simulink model "train_model_PetrFD"  (R2021b)
settings: Solver=FixedStepAuto  StartTime=0.0  StopTime=10  FixedStep=0.01  RelTol=1e-3
model workspace (MAT data in the model file):
  L = 50
  g = 9.8
undefined symbols (not defined in the file): l
libraries: simulink_extras x2
settings Model: Creator=PC  LastModifiedBy=PC

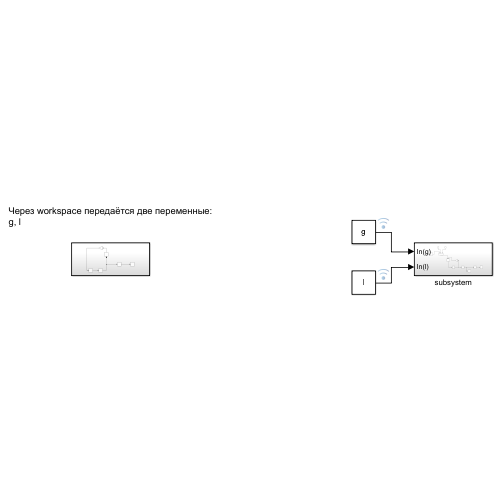
[thumbnail: Simulink's stored preview of the top-level diagram]
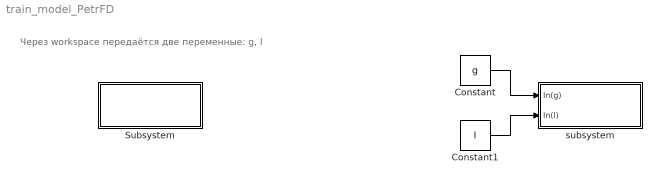
== system train_model_PetrFD ==
  note: Через workspace передаётся две переменные:
      | g, l
  Constant : Constant  Value=g
  Constant1 : Constant  Value=l
  Subsystem : Subsystem
  subsystem : Subsystem
  wires:
  Constant/1 -> subsystem/1(In(g))
  Constant1/1 -> subsystem/2(In(l))

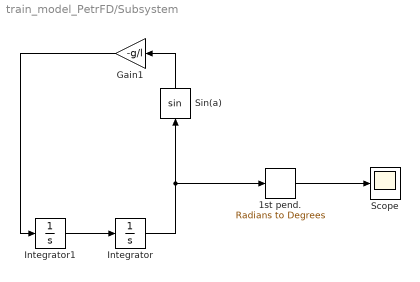
== system train_model_PetrFD/Subsystem ==
  1st pend. : simulink_extras/Transformations/Radians to Degrees
  Gain1 : Gain  Gain=-g/l
  Integrator : Integrator  InitialCondition=deg2rad(45)  AbsoluteTolerance=0.01
  Integrator1 : Integrator
  Scope : Scope
  Sin(a) : Trigonometry
  wires:
  1st pend./1 -> Scope/1
  Sin(a)/1 -> Gain1/1
  Integrator/1 -> 1st pend./1, Sin(a)/1
  Gain1/1 -> Integrator1/1
  Integrator1/1 -> Integrator/1

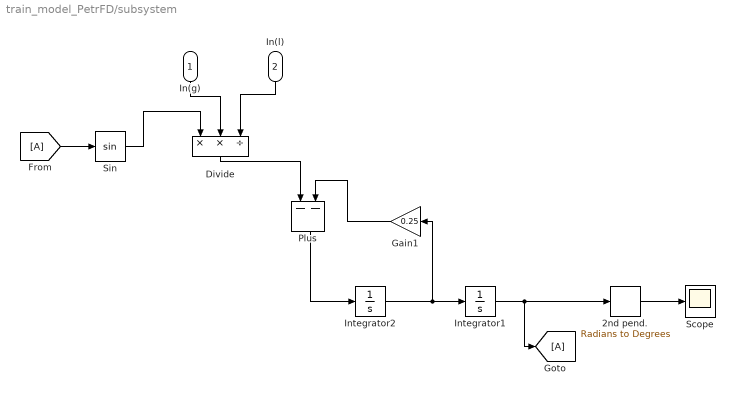
== system train_model_PetrFD/subsystem ==
  In(g) : Inport  OutDataTypeStr=double
  In(l) : Inport  Port=2  OutDataTypeStr=double
  2nd pend. : simulink_extras/Transformations/Radians to Degrees
  Divide : Product  Inputs=**/
  Gain1 : Gain  Gain=0.25
  Integrator1 : Integrator  InitialCondition=deg2rad(45)
  Integrator2 : Integrator
  Plus : Sum  Inputs=--
  Scope : Scope
  Sin : Trigonometry
  wires:
  Integrator2/1 -> Gain1/1, Integrator1/1
  Integrator1/1 -> 2nd pend./1, [A]
  Gain1/1 -> Plus/2
  Plus/1 -> Integrator2/1
  In(l)/1 -> Divide/3
  In(g)/1 -> Divide/2
  Sin/1 -> Divide/1
  Divide/1 -> Plus/1
  [A] -> Sin/1
  2nd pend./1 -> Scope/1
